simulink model "image_reject"  (R2014b)
settings: Solver=ode45  StartTime=0.0  StopTime=1  RelTol=1e-3
undefined symbols (not defined in the file or in its folder): fdesignblkfcn, gcbh
libraries: commrflib2 x1
settings Model: NumberOfSteps=100  Creator=Ben  LastModifiedBy=Ben

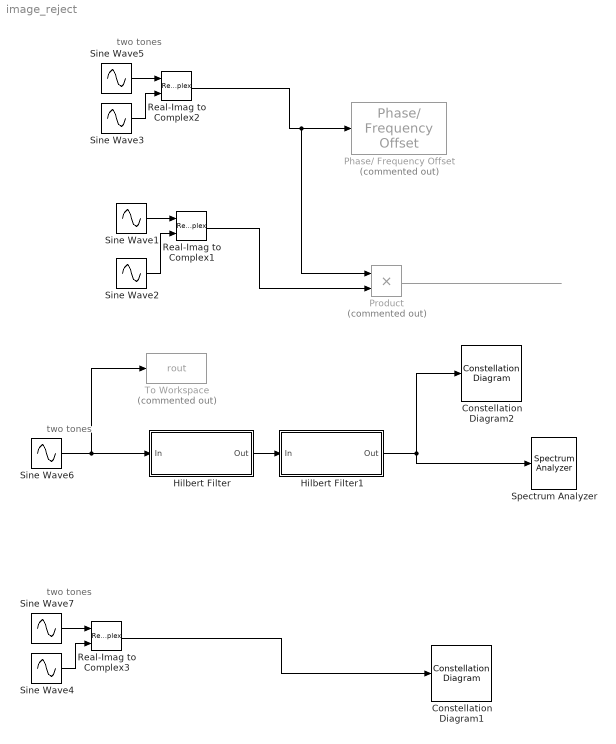
== system image_reject ==
  note: two tones
  note: two tones
  note: two tones
  Constellation Diagram1 : ConstellationDiagram
  Constellation Diagram2 : ConstellationDiagram
  Hilbert Filter : Subsystem  DialogController=fdesignblkfcn  InitFcn=fdesignblkfcn(gcbh, {'InitFcn'});  mask(Hilbert Filter){}
      mask help: Design a Hilbert filter
      settings: CopyFcn=fdesignblkfcn(gcbh, {'CopyFcn'});
      mask Help: helpview(mapfilelocation('dsp'), 'dsphilbertfilter');
      mask Display: disp('Hilbert')
  Hilbert Filter1 : Subsystem  DialogController=fdesignblkfcn  InitFcn=fdesignblkfcn(gcbh, {'InitFcn'});  mask(Hilbert Filter){}
      mask help: Design a Hilbert filter
      settings: CopyFcn=fdesignblkfcn(gcbh, {'CopyFcn'});
      mask Help: helpview(mapfilelocation('dsp'), 'dsphilbertfilter');
      mask Display: disp('Hilbert')
  Phase/ Frequency Offset : commrflib2/Phase// Frequency Offset  Commented=on  phaseOffset=0  freqPort=off  freqOffset=20000
  Product : Product  Commented=on
  Real-Imag to Complex1 : RealImagToComplex
  Real-Imag to Complex2 : RealImagToComplex
  Real-Imag to Complex3 : RealImagToComplex
  Sine Wave1 : Sin  Frequency=20000*2*pi  Phase=2*pi*90/360  SampleTime=2.00E-06
  Sine Wave2 : Sin  Frequency=20000*2*pi  SampleTime=2.00E-06
  Sine Wave{3..6} (4 alike) : Sin  Frequency=10*2*3.14*1000  SampleTime=2.00E-06
  Sine Wave7 : Sin  Frequency=10*2*3.14*1000  Phase=2*pi*90/360  SampleTime=2.00E-06
  Spectrum Analyzer : SpectrumAnalyzer
  To Workspace : ToWorkspace  Commented=on  VariableName=rout  SampleTime=-1
  wires:
  Sine Wave5/1 -> Real-Imag to Complex2/1
  Sine Wave1/1 -> Real-Imag to Complex1/1
  Real-Imag to Complex1/1 -> Product/2
  Real-Imag to Complex2/1 -> Product/1, Phase/ Frequency Offset/1
  Product/1 -> ?
  Sine Wave2/1 -> Real-Imag to Complex1/2
  Sine Wave3/1 -> Real-Imag to Complex2/2
  Sine Wave6/1 -> To Workspace/1, Hilbert Filter/1(In)
  Hilbert Filter/1(Out) -> Hilbert Filter1/1(In)
  Sine Wave7/1 -> Real-Imag to Complex3/1
  Sine Wave4/1 -> Real-Imag to Complex3/2
  Real-Imag to Complex3/1 -> Constellation Diagram1/1
  Hilbert Filter1/1(Out) -> Spectrum Analyzer/1, Constellation Diagram2/1

== system image_reject/Hilbert Filter ==
  In : Inport
  Generated Filter Block : Subsystem  Tag=FilterWizardSubSystem
  Out : Outport
  wires:
  Generated Filter Block/1(Output) -> Out/1
  In/1 -> Generated Filter Block/1(Input)

== system image_reject/Hilbert Filter1 ==
  In : Inport
  Generated Filter Block : Subsystem  Tag=FilterWizardSubSystem
  Out : Outport
  wires:
  Generated Filter Block/1(Output) -> Out/1
  In/1 -> Generated Filter Block/1(Input)

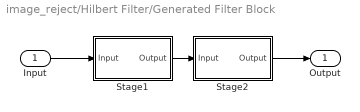
== system image_reject/Hilbert Filter/Generated Filter Block ==
  Input : Inport
  Stage1 : Subsystem  Tag=FilterWizardSubSystem
  Stage2 : Subsystem  Tag=FilterWizardSubSystem
      settings: ErrorFcn=dspFilterRealizedInBasicElemsAlgLoopErrFcnCallback
  Output : Outport
  wires:
  Input/1 -> Stage1/1(Input)
  Stage1/1(Output) -> Stage2/1(Input)
  Stage2/1(Output) -> Output/1

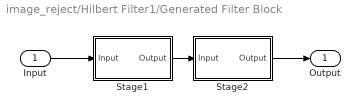
== system image_reject/Hilbert Filter1/Generated Filter Block ==
  Input : Inport
  Stage1 : Subsystem  Tag=FilterWizardSubSystem
  Stage2 : Subsystem  Tag=FilterWizardSubSystem
      settings: ErrorFcn=dspFilterRealizedInBasicElemsAlgLoopErrFcnCallback
  Output : Outport
  wires:
  Input/1 -> Stage1/1(Input)
  Stage1/1(Output) -> Stage2/1(Input)
  Stage2/1(Output) -> Output/1

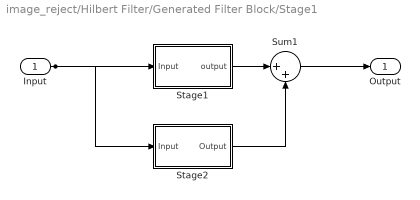
== system image_reject/Hilbert Filter/Generated Filter Block/Stage1 ==
  Input : Inport
  Stage1 : Subsystem  Tag=FilterWizardSubSystem
      settings: ErrorFcn=dspFilterRealizedInBasicElemsAlgLoopErrFcnCallback
  Stage2 : Subsystem  Tag=FilterWizardSubSystem
  Sum1 : Sum  Inputs=|++  RndMeth=Nearest  SaturateOnIntegerOverflow=on  OutDataTypeStr=Inherit: Same as first input
  Output : Outport
  wires:
  Stage1/1(output) -> Sum1/1
  Input/1 -> Stage1/1(Input), Stage2/1(Input)
  Stage2/1(Output) -> Sum1/2
  Sum1/1 -> Output/1

== system image_reject/Hilbert Filter/Generated Filter Block/Stage2 ==
  Input : Inport
  g(1) : Gain  Gain=0.5  ParamDataTypeStr=double  RndMeth=Nearest  SaturateOnIntegerOverflow=on  OutDataTypeStr=Inherit: Same as input
  Output : Outport
  wires:
  Input/1 -> g(1)/1
  g(1)/1 -> Output/1

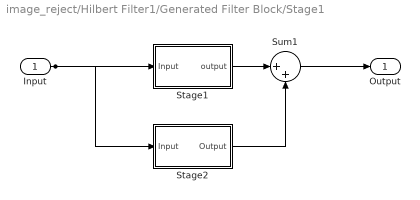
== system image_reject/Hilbert Filter1/Generated Filter Block/Stage1 ==
  Input : Inport
  Stage1 : Subsystem  Tag=FilterWizardSubSystem
      settings: ErrorFcn=dspFilterRealizedInBasicElemsAlgLoopErrFcnCallback
  Stage2 : Subsystem  Tag=FilterWizardSubSystem
  Sum1 : Sum  Inputs=|++  RndMeth=Nearest  SaturateOnIntegerOverflow=on  OutDataTypeStr=Inherit: Same as first input
  Output : Outport
  wires:
  Stage1/1(output) -> Sum1/1
  Input/1 -> Stage1/1(Input), Stage2/1(Input)
  Stage2/1(Output) -> Sum1/2
  Sum1/1 -> Output/1

== system image_reject/Hilbert Filter1/Generated Filter Block/Stage2 ==
  Input : Inport
  g(1) : Gain  Gain=0.5  ParamDataTypeStr=double  RndMeth=Nearest  SaturateOnIntegerOverflow=on  OutDataTypeStr=Inherit: Same as input
  Output : Outport
  wires:
  Input/1 -> g(1)/1
  g(1)/1 -> Output/1

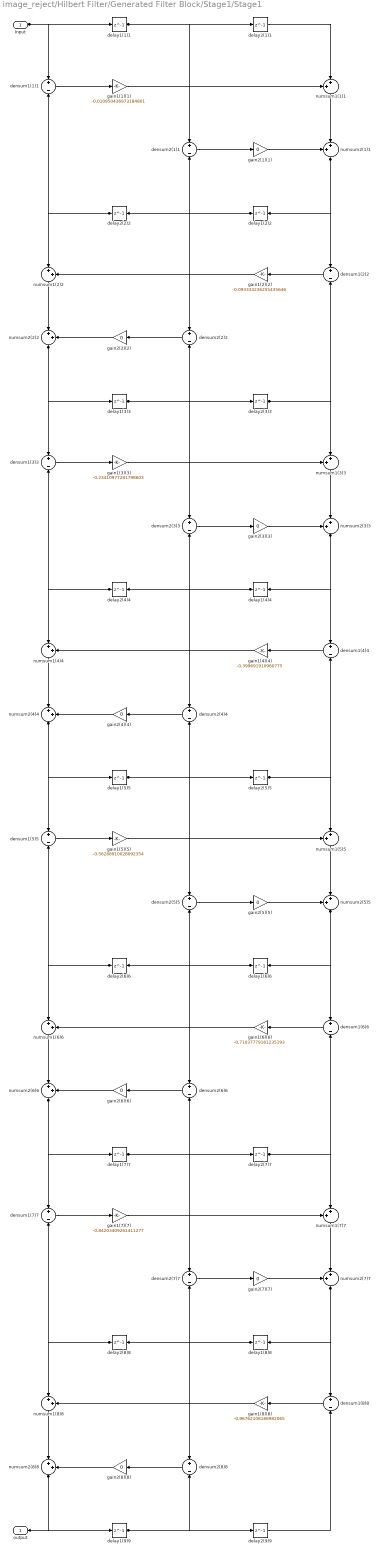
== system image_reject/Hilbert Filter/Generated Filter Block/Stage1/Stage1 ==
  Input : Inport
  delay1(1)1 : Delay  DelayLength=1  InitialCondition=0
  delay1(2)2 : Delay  DelayLength=1  InitialCondition=0
  delay1(3)3 : Delay  DelayLength=1  InitialCondition=0
  delay1(4)4 : Delay  DelayLength=1  InitialCondition=0
  delay1(5)5 : Delay  DelayLength=1  InitialCondition=0
  delay1(6)6 : Delay  DelayLength=1  InitialCondition=0
  delay1(7)7 : Delay  DelayLength=1  InitialCondition=0
  delay1(8)8 : Delay  DelayLength=1  InitialCondition=0
  delay1(9)9 : Delay  DelayLength=1  InitialCondition=0
  delay2(1)1 : Delay  DelayLength=1  InitialCondition=0
  delay2(2)2 : Delay  DelayLength=1  InitialCondition=0
  delay2(3)3 : Delay  DelayLength=1  InitialCondition=0
  delay2(4)4 : Delay  DelayLength=1  InitialCondition=0
  delay2(5)5 : Delay  DelayLength=1  InitialCondition=0
  delay2(6)6 : Delay  DelayLength=1  InitialCondition=0
  delay2(7)7 : Delay  DelayLength=1  InitialCondition=0
  delay2(8)8 : Delay  DelayLength=1  InitialCondition=0
  delay2(9)9 : Delay  DelayLength=1  InitialCondition=0
  densum1(1)1 : Sum  Inputs=+|-  RndMeth=Nearest  SaturateOnIntegerOverflow=on  OutDataTypeStr=Inherit: Same as first input
  densum1(2)2 : Sum  Inputs=+|-  RndMeth=Nearest  SaturateOnIntegerOverflow=on  OutDataTypeStr=Inherit: Same as first input
  densum1(3)3 : Sum  Inputs=+|-  RndMeth=Nearest  SaturateOnIntegerOverflow=on  OutDataTypeStr=Inherit: Same as first input
  densum1(4)4 : Sum  Inputs=+|-  RndMeth=Nearest  SaturateOnIntegerOverflow=on  OutDataTypeStr=Inherit: Same as first input
  densum1(5)5 : Sum  Inputs=+|-  RndMeth=Nearest  SaturateOnIntegerOverflow=on  OutDataTypeStr=Inherit: Same as first input
  densum1(6)6 : Sum  Inputs=+|-  RndMeth=Nearest  SaturateOnIntegerOverflow=on  OutDataTypeStr=Inherit: Same as first input
  densum1(7)7 : Sum  Inputs=+|-  RndMeth=Nearest  SaturateOnIntegerOverflow=on  OutDataTypeStr=Inherit: Same as first input
  densum1(8)8 : Sum  Inputs=+|-  RndMeth=Nearest  SaturateOnIntegerOverflow=on  OutDataTypeStr=Inherit: Same as first input
  densum2(1)1 : Sum  Inputs=+|-  RndMeth=Nearest  SaturateOnIntegerOverflow=on  OutDataTypeStr=Inherit: Same as first input
  densum2(2)2 : Sum  Inputs=+|-  RndMeth=Nearest  SaturateOnIntegerOverflow=on  OutDataTypeStr=Inherit: Same as first input
  densum2(3)3 : Sum  Inputs=+|-  RndMeth=Nearest  SaturateOnIntegerOverflow=on  OutDataTypeStr=Inherit: Same as first input
  densum2(4)4 : Sum  Inputs=+|-  RndMeth=Nearest  SaturateOnIntegerOverflow=on  OutDataTypeStr=Inherit: Same as first input
  densum2(5)5 : Sum  Inputs=+|-  RndMeth=Nearest  SaturateOnIntegerOverflow=on  OutDataTypeStr=Inherit: Same as first input
  densum2(6)6 : Sum  Inputs=+|-  RndMeth=Nearest  SaturateOnIntegerOverflow=on  OutDataTypeStr=Inherit: Same as first input
  densum2(7)7 : Sum  Inputs=+|-  RndMeth=Nearest  SaturateOnIntegerOverflow=on  OutDataTypeStr=Inherit: Same as first input
  densum2(8)8 : Sum  Inputs=+|-  RndMeth=Nearest  SaturateOnIntegerOverflow=on  OutDataTypeStr=Inherit: Same as first input
  gain1(1)(1) : Gain  Gain=-0.010950436973184801  ParamDataTypeStr=double  RndMeth=Nearest  SaturateOnIntegerOverflow=on  OutDataTypeStr=Inherit: Same as input
  gain1(2)(2) : Gain  Gain=-0.093334236255435646  ParamDataTypeStr=double  RndMeth=Nearest  SaturateOnIntegerOverflow=on  OutDataTypeStr=Inherit: Same as input
  gain1(3)(3) : Gain  Gain=-0.23410977281798603  ParamDataTypeStr=double  RndMeth=Nearest  SaturateOnIntegerOverflow=on  OutDataTypeStr=Inherit: Same as input
  gain1(4)(4) : Gain  Gain=-0.399691910960775  ParamDataTypeStr=double  RndMeth=Nearest  SaturateOnIntegerOverflow=on  OutDataTypeStr=Inherit: Same as input
  gain1(5)(5) : Gain  Gain=-0.56288910028092354  ParamDataTypeStr=double  RndMeth=Nearest  SaturateOnIntegerOverflow=on  OutDataTypeStr=Inherit: Same as input
  gain1(6)(6) : Gain  Gain=-0.71037779161235193  ParamDataTypeStr=double  RndMeth=Nearest  SaturateOnIntegerOverflow=on  OutDataTypeStr=Inherit: Same as input
  gain1(7)(7) : Gain  Gain=-0.84203409261411277  ParamDataTypeStr=double  RndMeth=Nearest  SaturateOnIntegerOverflow=on  OutDataTypeStr=Inherit: Same as input
  gain1(8)(8) : Gain  Gain=-0.96762108186982065  ParamDataTypeStr=double  RndMeth=Nearest  SaturateOnIntegerOverflow=on  OutDataTypeStr=Inherit: Same as input
  gain2(1)(1) : Gain  Gain=0  ParamDataTypeStr=double  RndMeth=Nearest  SaturateOnIntegerOverflow=on  OutDataTypeStr=Inherit: Same as input
  gain2(2)(2) : Gain  Gain=0  ParamDataTypeStr=double  RndMeth=Nearest  SaturateOnIntegerOverflow=on  OutDataTypeStr=Inherit: Same as input
  gain2(3)(3) : Gain  Gain=0  ParamDataTypeStr=double  RndMeth=Nearest  SaturateOnIntegerOverflow=on  OutDataTypeStr=Inherit: Same as input
  gain2(4)(4) : Gain  Gain=0  ParamDataTypeStr=double  RndMeth=Nearest  SaturateOnIntegerOverflow=on  OutDataTypeStr=Inherit: Same as input
  gain2(5)(5) : Gain  Gain=0  ParamDataTypeStr=double  RndMeth=Nearest  SaturateOnIntegerOverflow=on  OutDataTypeStr=Inherit: Same as input
  gain2(6)(6) : Gain  Gain=0  ParamDataTypeStr=double  RndMeth=Nearest  SaturateOnIntegerOverflow=on  OutDataTypeStr=Inherit: Same as input
  gain2(7)(7) : Gain  Gain=0  ParamDataTypeStr=double  RndMeth=Nearest  SaturateOnIntegerOverflow=on  OutDataTypeStr=Inherit: Same as input
  gain2(8)(8) : Gain  Gain=0  ParamDataTypeStr=double  RndMeth=Nearest  SaturateOnIntegerOverflow=on  OutDataTypeStr=Inherit: Same as input
  numsum1(1)1 : Sum  Inputs=++|  RndMeth=Nearest  SaturateOnIntegerOverflow=on  OutDataTypeStr=Inherit: Same as first input
  numsum1(2)2 : Sum  Inputs=|++  RndMeth=Nearest  SaturateOnIntegerOverflow=on  OutDataTypeStr=Inherit: Same as first input
  numsum1(3)3 : Sum  Inputs=++|  RndMeth=Nearest  SaturateOnIntegerOverflow=on  OutDataTypeStr=Inherit: Same as first input
  numsum1(4)4 : Sum  Inputs=|++  RndMeth=Nearest  SaturateOnIntegerOverflow=on  OutDataTypeStr=Inherit: Same as first input
  numsum1(5)5 : Sum  Inputs=++|  RndMeth=Nearest  SaturateOnIntegerOverflow=on  OutDataTypeStr=Inherit: Same as first input
  numsum1(6)6 : Sum  Inputs=|++  RndMeth=Nearest  SaturateOnIntegerOverflow=on  OutDataTypeStr=Inherit: Same as first input
  numsum1(7)7 : Sum  Inputs=++|  RndMeth=Nearest  SaturateOnIntegerOverflow=on  OutDataTypeStr=Inherit: Same as first input
  numsum1(8)8 : Sum  Inputs=|++  RndMeth=Nearest  SaturateOnIntegerOverflow=on  OutDataTypeStr=Inherit: Same as first input
  numsum2(1)1 : Sum  Inputs=++|  RndMeth=Nearest  SaturateOnIntegerOverflow=on  OutDataTypeStr=Inherit: Same as first input
  numsum2(2)2 : Sum  Inputs=|++  RndMeth=Nearest  SaturateOnIntegerOverflow=on  OutDataTypeStr=Inherit: Same as first input
  numsum2(3)3 : Sum  Inputs=++|  RndMeth=Nearest  SaturateOnIntegerOverflow=on  OutDataTypeStr=Inherit: Same as first input
  numsum2(4)4 : Sum  Inputs=|++  RndMeth=Nearest  SaturateOnIntegerOverflow=on  OutDataTypeStr=Inherit: Same as first input
  numsum2(5)5 : Sum  Inputs=++|  RndMeth=Nearest  SaturateOnIntegerOverflow=on  OutDataTypeStr=Inherit: Same as first input
  numsum2(6)6 : Sum  Inputs=|++  RndMeth=Nearest  SaturateOnIntegerOverflow=on  OutDataTypeStr=Inherit: Same as first input
  numsum2(7)7 : Sum  Inputs=++|  RndMeth=Nearest  SaturateOnIntegerOverflow=on  OutDataTypeStr=Inherit: Same as first input
  numsum2(8)8 : Sum  Inputs=|++  RndMeth=Nearest  SaturateOnIntegerOverflow=on  OutDataTypeStr=Inherit: Same as first input
  output : Outport
  wires:
  delay1(1)1/1 -> delay2(1)1/1, densum2(1)1/1
  delay2(1)1/1 -> numsum1(1)1/2
  densum1(1)1/1 -> gain1(1)(1)/1
  gain1(1)(1)/1 -> numsum1(1)1/1
  numsum1(1)1/1 -> numsum2(1)1/2
  densum2(1)1/1 -> gain2(1)(1)/1
  gain2(1)(1)/1 -> numsum2(1)1/1
  numsum2(1)1/1 -> delay1(2)2/1, densum1(2)2/1
  Input/1 -> delay1(1)1/1, densum1(1)1/1
  delay1(2)2/1 -> delay2(2)2/1, densum2(2)2/1, densum2(1)1/2
  delay2(2)2/1 -> numsum1(2)2/1, densum1(1)1/2
  densum1(2)2/1 -> gain1(2)(2)/1
  gain1(2)(2)/1 -> numsum1(2)2/2
  numsum1(2)2/1 -> numsum2(2)2/1
  densum2(2)2/1 -> gain2(2)(2)/1
  gain2(2)(2)/1 -> numsum2(2)2/2
  numsum2(2)2/1 -> delay1(3)3/1, densum1(3)3/1
  delay1(3)3/1 -> delay2(3)3/1, densum2(3)3/1, densum2(2)2/2
  delay2(3)3/1 -> numsum1(3)3/2, densum1(2)2/2
  densum1(3)3/1 -> gain1(3)(3)/1
  gain1(3)(3)/1 -> numsum1(3)3/1
  numsum1(3)3/1 -> numsum2(3)3/2
  densum2(3)3/1 -> gain2(3)(3)/1
  gain2(3)(3)/1 -> numsum2(3)3/1
  numsum2(3)3/1 -> delay1(4)4/1, densum1(4)4/1
  delay1(4)4/1 -> delay2(4)4/1, densum2(4)4/1, densum2(3)3/2
  delay2(4)4/1 -> numsum1(4)4/1, densum1(3)3/2
  densum1(4)4/1 -> gain1(4)(4)/1
  gain1(4)(4)/1 -> numsum1(4)4/2
  numsum1(4)4/1 -> numsum2(4)4/1
  densum2(4)4/1 -> gain2(4)(4)/1
  gain2(4)(4)/1 -> numsum2(4)4/2
  numsum2(4)4/1 -> delay1(5)5/1, densum1(5)5/1
  delay1(5)5/1 -> delay2(5)5/1, densum2(5)5/1, densum2(4)4/2
  delay2(5)5/1 -> numsum1(5)5/2, densum1(4)4/2
  densum1(5)5/1 -> gain1(5)(5)/1
  gain1(5)(5)/1 -> numsum1(5)5/1
  numsum1(5)5/1 -> numsum2(5)5/2
  densum2(5)5/1 -> gain2(5)(5)/1
  gain2(5)(5)/1 -> numsum2(5)5/1
  numsum2(5)5/1 -> delay1(6)6/1, densum1(6)6/1
  delay1(6)6/1 -> delay2(6)6/1, densum2(6)6/1, densum2(5)5/2
  delay2(6)6/1 -> numsum1(6)6/1, densum1(5)5/2
  densum1(6)6/1 -> gain1(6)(6)/1
  gain1(6)(6)/1 -> numsum1(6)6/2
  numsum1(6)6/1 -> numsum2(6)6/1
  densum2(6)6/1 -> gain2(6)(6)/1
  gain2(6)(6)/1 -> numsum2(6)6/2
  numsum2(6)6/1 -> delay1(7)7/1, densum1(7)7/1
  delay1(7)7/1 -> delay2(7)7/1, densum2(7)7/1, densum2(6)6/2
  delay2(7)7/1 -> numsum1(7)7/2, densum1(6)6/2
  densum1(7)7/1 -> gain1(7)(7)/1
  gain1(7)(7)/1 -> numsum1(7)7/1
  numsum1(7)7/1 -> numsum2(7)7/2
  densum2(7)7/1 -> gain2(7)(7)/1
  gain2(7)(7)/1 -> numsum2(7)7/1
  numsum2(7)7/1 -> delay1(8)8/1, densum1(8)8/1
  delay1(8)8/1 -> delay2(8)8/1, densum2(8)8/1, densum2(7)7/2
  delay2(8)8/1 -> numsum1(8)8/1, densum1(7)7/2
  densum1(8)8/1 -> gain1(8)(8)/1
  gain1(8)(8)/1 -> numsum1(8)8/2
  numsum1(8)8/1 -> numsum2(8)8/1
  densum2(8)8/1 -> gain2(8)(8)/1
  gain2(8)(8)/1 -> numsum2(8)8/2
  numsum2(8)8/1 -> delay1(9)9/1, output/1
  delay1(9)9/1 -> delay2(9)9/1, densum2(8)8/2
  delay2(9)9/1 -> densum1(8)8/2

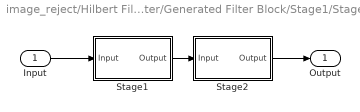
== system image_reject/Hilbert Filter/Generated Filter Block/Stage1/Stage2 ==
  Input : Inport
  Stage1 : Subsystem  Tag=FilterWizardSubSystem
      settings: ErrorFcn=dspFilterRealizedInBasicElemsAlgLoopErrFcnCallback
  Stage2 : Subsystem  Tag=FilterWizardSubSystem
  Output : Outport
  wires:
  Input/1 -> Stage1/1(Input)
  Stage1/1(Output) -> Stage2/1(Input)
  Stage2/1(Output) -> Output/1

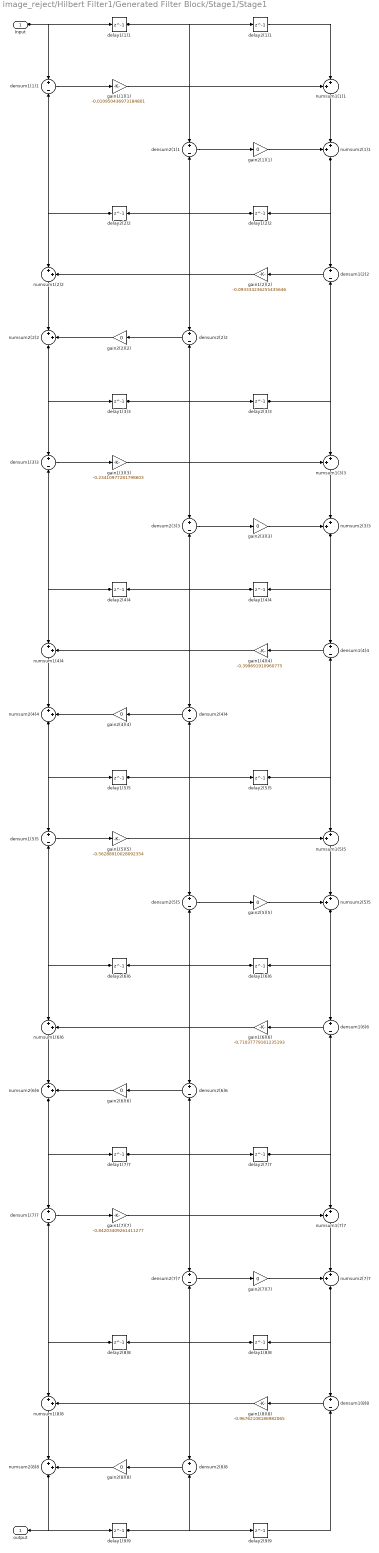
== system image_reject/Hilbert Filter1/Generated Filter Block/Stage1/Stage1 ==
  Input : Inport
  delay1(1)1 : Delay  DelayLength=1  InitialCondition=0
  delay1(2)2 : Delay  DelayLength=1  InitialCondition=0
  delay1(3)3 : Delay  DelayLength=1  InitialCondition=0
  delay1(4)4 : Delay  DelayLength=1  InitialCondition=0
  delay1(5)5 : Delay  DelayLength=1  InitialCondition=0
  delay1(6)6 : Delay  DelayLength=1  InitialCondition=0
  delay1(7)7 : Delay  DelayLength=1  InitialCondition=0
  delay1(8)8 : Delay  DelayLength=1  InitialCondition=0
  delay1(9)9 : Delay  DelayLength=1  InitialCondition=0
  delay2(1)1 : Delay  DelayLength=1  InitialCondition=0
  delay2(2)2 : Delay  DelayLength=1  InitialCondition=0
  delay2(3)3 : Delay  DelayLength=1  InitialCondition=0
  delay2(4)4 : Delay  DelayLength=1  InitialCondition=0
  delay2(5)5 : Delay  DelayLength=1  InitialCondition=0
  delay2(6)6 : Delay  DelayLength=1  InitialCondition=0
  delay2(7)7 : Delay  DelayLength=1  InitialCondition=0
  delay2(8)8 : Delay  DelayLength=1  InitialCondition=0
  delay2(9)9 : Delay  DelayLength=1  InitialCondition=0
  densum1(1)1 : Sum  Inputs=+|-  RndMeth=Nearest  SaturateOnIntegerOverflow=on  OutDataTypeStr=Inherit: Same as first input
  densum1(2)2 : Sum  Inputs=+|-  RndMeth=Nearest  SaturateOnIntegerOverflow=on  OutDataTypeStr=Inherit: Same as first input
  densum1(3)3 : Sum  Inputs=+|-  RndMeth=Nearest  SaturateOnIntegerOverflow=on  OutDataTypeStr=Inherit: Same as first input
  densum1(4)4 : Sum  Inputs=+|-  RndMeth=Nearest  SaturateOnIntegerOverflow=on  OutDataTypeStr=Inherit: Same as first input
  densum1(5)5 : Sum  Inputs=+|-  RndMeth=Nearest  SaturateOnIntegerOverflow=on  OutDataTypeStr=Inherit: Same as first input
  densum1(6)6 : Sum  Inputs=+|-  RndMeth=Nearest  SaturateOnIntegerOverflow=on  OutDataTypeStr=Inherit: Same as first input
  densum1(7)7 : Sum  Inputs=+|-  RndMeth=Nearest  SaturateOnIntegerOverflow=on  OutDataTypeStr=Inherit: Same as first input
  densum1(8)8 : Sum  Inputs=+|-  RndMeth=Nearest  SaturateOnIntegerOverflow=on  OutDataTypeStr=Inherit: Same as first input
  densum2(1)1 : Sum  Inputs=+|-  RndMeth=Nearest  SaturateOnIntegerOverflow=on  OutDataTypeStr=Inherit: Same as first input
  densum2(2)2 : Sum  Inputs=+|-  RndMeth=Nearest  SaturateOnIntegerOverflow=on  OutDataTypeStr=Inherit: Same as first input
  densum2(3)3 : Sum  Inputs=+|-  RndMeth=Nearest  SaturateOnIntegerOverflow=on  OutDataTypeStr=Inherit: Same as first input
  densum2(4)4 : Sum  Inputs=+|-  RndMeth=Nearest  SaturateOnIntegerOverflow=on  OutDataTypeStr=Inherit: Same as first input
  densum2(5)5 : Sum  Inputs=+|-  RndMeth=Nearest  SaturateOnIntegerOverflow=on  OutDataTypeStr=Inherit: Same as first input
  densum2(6)6 : Sum  Inputs=+|-  RndMeth=Nearest  SaturateOnIntegerOverflow=on  OutDataTypeStr=Inherit: Same as first input
  densum2(7)7 : Sum  Inputs=+|-  RndMeth=Nearest  SaturateOnIntegerOverflow=on  OutDataTypeStr=Inherit: Same as first input
  densum2(8)8 : Sum  Inputs=+|-  RndMeth=Nearest  SaturateOnIntegerOverflow=on  OutDataTypeStr=Inherit: Same as first input
  gain1(1)(1) : Gain  Gain=-0.010950436973184801  ParamDataTypeStr=double  RndMeth=Nearest  SaturateOnIntegerOverflow=on  OutDataTypeStr=Inherit: Same as input
  gain1(2)(2) : Gain  Gain=-0.093334236255435646  ParamDataTypeStr=double  RndMeth=Nearest  SaturateOnIntegerOverflow=on  OutDataTypeStr=Inherit: Same as input
  gain1(3)(3) : Gain  Gain=-0.23410977281798603  ParamDataTypeStr=double  RndMeth=Nearest  SaturateOnIntegerOverflow=on  OutDataTypeStr=Inherit: Same as input
  gain1(4)(4) : Gain  Gain=-0.399691910960775  ParamDataTypeStr=double  RndMeth=Nearest  SaturateOnIntegerOverflow=on  OutDataTypeStr=Inherit: Same as input
  gain1(5)(5) : Gain  Gain=-0.56288910028092354  ParamDataTypeStr=double  RndMeth=Nearest  SaturateOnIntegerOverflow=on  OutDataTypeStr=Inherit: Same as input
  gain1(6)(6) : Gain  Gain=-0.71037779161235193  ParamDataTypeStr=double  RndMeth=Nearest  SaturateOnIntegerOverflow=on  OutDataTypeStr=Inherit: Same as input
  gain1(7)(7) : Gain  Gain=-0.84203409261411277  ParamDataTypeStr=double  RndMeth=Nearest  SaturateOnIntegerOverflow=on  OutDataTypeStr=Inherit: Same as input
  gain1(8)(8) : Gain  Gain=-0.96762108186982065  ParamDataTypeStr=double  RndMeth=Nearest  SaturateOnIntegerOverflow=on  OutDataTypeStr=Inherit: Same as input
  gain2(1)(1) : Gain  Gain=0  ParamDataTypeStr=double  RndMeth=Nearest  SaturateOnIntegerOverflow=on  OutDataTypeStr=Inherit: Same as input
  gain2(2)(2) : Gain  Gain=0  ParamDataTypeStr=double  RndMeth=Nearest  SaturateOnIntegerOverflow=on  OutDataTypeStr=Inherit: Same as input
  gain2(3)(3) : Gain  Gain=0  ParamDataTypeStr=double  RndMeth=Nearest  SaturateOnIntegerOverflow=on  OutDataTypeStr=Inherit: Same as input
  gain2(4)(4) : Gain  Gain=0  ParamDataTypeStr=double  RndMeth=Nearest  SaturateOnIntegerOverflow=on  OutDataTypeStr=Inherit: Same as input
  gain2(5)(5) : Gain  Gain=0  ParamDataTypeStr=double  RndMeth=Nearest  SaturateOnIntegerOverflow=on  OutDataTypeStr=Inherit: Same as input
  gain2(6)(6) : Gain  Gain=0  ParamDataTypeStr=double  RndMeth=Nearest  SaturateOnIntegerOverflow=on  OutDataTypeStr=Inherit: Same as input
  gain2(7)(7) : Gain  Gain=0  ParamDataTypeStr=double  RndMeth=Nearest  SaturateOnIntegerOverflow=on  OutDataTypeStr=Inherit: Same as input
  gain2(8)(8) : Gain  Gain=0  ParamDataTypeStr=double  RndMeth=Nearest  SaturateOnIntegerOverflow=on  OutDataTypeStr=Inherit: Same as input
  numsum1(1)1 : Sum  Inputs=++|  RndMeth=Nearest  SaturateOnIntegerOverflow=on  OutDataTypeStr=Inherit: Same as first input
  numsum1(2)2 : Sum  Inputs=|++  RndMeth=Nearest  SaturateOnIntegerOverflow=on  OutDataTypeStr=Inherit: Same as first input
  numsum1(3)3 : Sum  Inputs=++|  RndMeth=Nearest  SaturateOnIntegerOverflow=on  OutDataTypeStr=Inherit: Same as first input
  numsum1(4)4 : Sum  Inputs=|++  RndMeth=Nearest  SaturateOnIntegerOverflow=on  OutDataTypeStr=Inherit: Same as first input
  numsum1(5)5 : Sum  Inputs=++|  RndMeth=Nearest  SaturateOnIntegerOverflow=on  OutDataTypeStr=Inherit: Same as first input
  numsum1(6)6 : Sum  Inputs=|++  RndMeth=Nearest  SaturateOnIntegerOverflow=on  OutDataTypeStr=Inherit: Same as first input
  numsum1(7)7 : Sum  Inputs=++|  RndMeth=Nearest  SaturateOnIntegerOverflow=on  OutDataTypeStr=Inherit: Same as first input
  numsum1(8)8 : Sum  Inputs=|++  RndMeth=Nearest  SaturateOnIntegerOverflow=on  OutDataTypeStr=Inherit: Same as first input
  numsum2(1)1 : Sum  Inputs=++|  RndMeth=Nearest  SaturateOnIntegerOverflow=on  OutDataTypeStr=Inherit: Same as first input
  numsum2(2)2 : Sum  Inputs=|++  RndMeth=Nearest  SaturateOnIntegerOverflow=on  OutDataTypeStr=Inherit: Same as first input
  numsum2(3)3 : Sum  Inputs=++|  RndMeth=Nearest  SaturateOnIntegerOverflow=on  OutDataTypeStr=Inherit: Same as first input
  numsum2(4)4 : Sum  Inputs=|++  RndMeth=Nearest  SaturateOnIntegerOverflow=on  OutDataTypeStr=Inherit: Same as first input
  numsum2(5)5 : Sum  Inputs=++|  RndMeth=Nearest  SaturateOnIntegerOverflow=on  OutDataTypeStr=Inherit: Same as first input
  numsum2(6)6 : Sum  Inputs=|++  RndMeth=Nearest  SaturateOnIntegerOverflow=on  OutDataTypeStr=Inherit: Same as first input
  numsum2(7)7 : Sum  Inputs=++|  RndMeth=Nearest  SaturateOnIntegerOverflow=on  OutDataTypeStr=Inherit: Same as first input
  numsum2(8)8 : Sum  Inputs=|++  RndMeth=Nearest  SaturateOnIntegerOverflow=on  OutDataTypeStr=Inherit: Same as first input
  output : Outport
  wires:
  delay1(1)1/1 -> delay2(1)1/1, densum2(1)1/1
  delay2(1)1/1 -> numsum1(1)1/2
  densum1(1)1/1 -> gain1(1)(1)/1
  gain1(1)(1)/1 -> numsum1(1)1/1
  numsum1(1)1/1 -> numsum2(1)1/2
  densum2(1)1/1 -> gain2(1)(1)/1
  gain2(1)(1)/1 -> numsum2(1)1/1
  numsum2(1)1/1 -> delay1(2)2/1, densum1(2)2/1
  Input/1 -> delay1(1)1/1, densum1(1)1/1
  delay1(2)2/1 -> delay2(2)2/1, densum2(2)2/1, densum2(1)1/2
  delay2(2)2/1 -> numsum1(2)2/1, densum1(1)1/2
  densum1(2)2/1 -> gain1(2)(2)/1
  gain1(2)(2)/1 -> numsum1(2)2/2
  numsum1(2)2/1 -> numsum2(2)2/1
  densum2(2)2/1 -> gain2(2)(2)/1
  gain2(2)(2)/1 -> numsum2(2)2/2
  numsum2(2)2/1 -> delay1(3)3/1, densum1(3)3/1
  delay1(3)3/1 -> delay2(3)3/1, densum2(3)3/1, densum2(2)2/2
  delay2(3)3/1 -> numsum1(3)3/2, densum1(2)2/2
  densum1(3)3/1 -> gain1(3)(3)/1
  gain1(3)(3)/1 -> numsum1(3)3/1
  numsum1(3)3/1 -> numsum2(3)3/2
  densum2(3)3/1 -> gain2(3)(3)/1
  gain2(3)(3)/1 -> numsum2(3)3/1
  numsum2(3)3/1 -> delay1(4)4/1, densum1(4)4/1
  delay1(4)4/1 -> delay2(4)4/1, densum2(4)4/1, densum2(3)3/2
  delay2(4)4/1 -> numsum1(4)4/1, densum1(3)3/2
  densum1(4)4/1 -> gain1(4)(4)/1
  gain1(4)(4)/1 -> numsum1(4)4/2
  numsum1(4)4/1 -> numsum2(4)4/1
  densum2(4)4/1 -> gain2(4)(4)/1
  gain2(4)(4)/1 -> numsum2(4)4/2
  numsum2(4)4/1 -> delay1(5)5/1, densum1(5)5/1
  delay1(5)5/1 -> delay2(5)5/1, densum2(5)5/1, densum2(4)4/2
  delay2(5)5/1 -> numsum1(5)5/2, densum1(4)4/2
  densum1(5)5/1 -> gain1(5)(5)/1
  gain1(5)(5)/1 -> numsum1(5)5/1
  numsum1(5)5/1 -> numsum2(5)5/2
  densum2(5)5/1 -> gain2(5)(5)/1
  gain2(5)(5)/1 -> numsum2(5)5/1
  numsum2(5)5/1 -> delay1(6)6/1, densum1(6)6/1
  delay1(6)6/1 -> delay2(6)6/1, densum2(6)6/1, densum2(5)5/2
  delay2(6)6/1 -> numsum1(6)6/1, densum1(5)5/2
  densum1(6)6/1 -> gain1(6)(6)/1
  gain1(6)(6)/1 -> numsum1(6)6/2
  numsum1(6)6/1 -> numsum2(6)6/1
  densum2(6)6/1 -> gain2(6)(6)/1
  gain2(6)(6)/1 -> numsum2(6)6/2
  numsum2(6)6/1 -> delay1(7)7/1, densum1(7)7/1
  delay1(7)7/1 -> delay2(7)7/1, densum2(7)7/1, densum2(6)6/2
  delay2(7)7/1 -> numsum1(7)7/2, densum1(6)6/2
  densum1(7)7/1 -> gain1(7)(7)/1
  gain1(7)(7)/1 -> numsum1(7)7/1
  numsum1(7)7/1 -> numsum2(7)7/2
  densum2(7)7/1 -> gain2(7)(7)/1
  gain2(7)(7)/1 -> numsum2(7)7/1
  numsum2(7)7/1 -> delay1(8)8/1, densum1(8)8/1
  delay1(8)8/1 -> delay2(8)8/1, densum2(8)8/1, densum2(7)7/2
  delay2(8)8/1 -> numsum1(8)8/1, densum1(7)7/2
  densum1(8)8/1 -> gain1(8)(8)/1
  gain1(8)(8)/1 -> numsum1(8)8/2
  numsum1(8)8/1 -> numsum2(8)8/1
  densum2(8)8/1 -> gain2(8)(8)/1
  gain2(8)(8)/1 -> numsum2(8)8/2
  numsum2(8)8/1 -> delay1(9)9/1, output/1
  delay1(9)9/1 -> delay2(9)9/1, densum2(8)8/2
  delay2(9)9/1 -> densum1(8)8/2

== system image_reject/Hilbert Filter1/Generated Filter Block/Stage1/Stage2 ==
  Input : Inport
  Stage1 : Subsystem  Tag=FilterWizardSubSystem
      settings: ErrorFcn=dspFilterRealizedInBasicElemsAlgLoopErrFcnCallback
  Stage2 : Subsystem  Tag=FilterWizardSubSystem
  Output : Outport
  wires:
  Input/1 -> Stage1/1(Input)
  Stage1/1(Output) -> Stage2/1(Input)
  Stage2/1(Output) -> Output/1

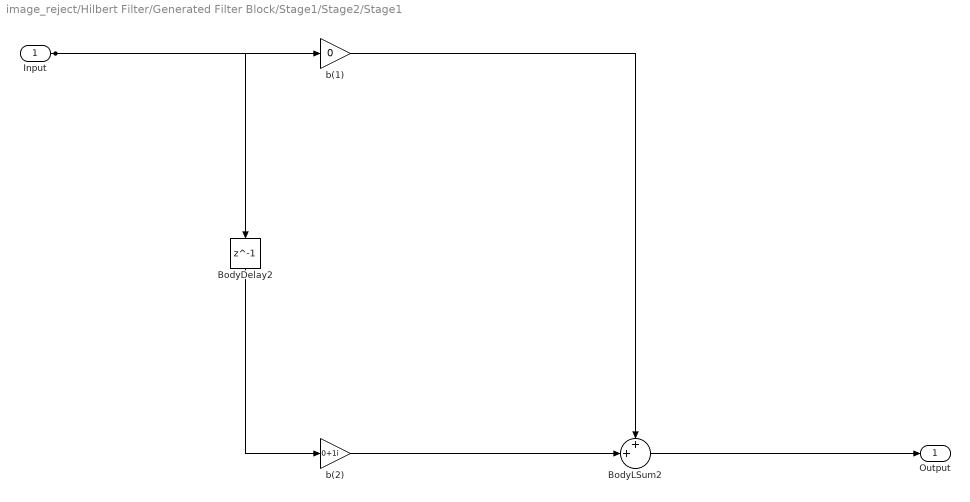
== system image_reject/Hilbert Filter/Generated Filter Block/Stage1/Stage2/Stage1 ==
  Input : Inport
  BodyDelay2 : Delay  DelayLength=1  InitialCondition=0
  BodyLSum2 : Sum  Inputs=++|  RndMeth=Nearest  SaturateOnIntegerOverflow=on  OutDataTypeStr=Inherit: Same as first input
  b(1) : Gain  Gain=0  ParamDataTypeStr=double  RndMeth=Nearest  SaturateOnIntegerOverflow=on  OutDataTypeStr=Inherit: Same as input
  b(2) : Gain  Gain=0+1i  ParamDataTypeStr=double  RndMeth=Nearest  SaturateOnIntegerOverflow=on  OutDataTypeStr=Inherit: Same as input
  Output : Outport
  wires:
  Input/1 -> b(1)/1, BodyDelay2/1
  b(1)/1 -> BodyLSum2/1
  BodyDelay2/1 -> b(2)/1
  b(2)/1 -> BodyLSum2/2
  BodyLSum2/1 -> Output/1

== system image_reject/Hilbert Filter/Generated Filter Block/Stage1/Stage2/Stage2 ==
  Input : Inport
  Stage1 : Subsystem  Tag=FilterWizardSubSystem
      settings: ErrorFcn=dspFilterRealizedInBasicElemsAlgLoopErrFcnCallback
  Stage2 : Subsystem  Tag=FilterWizardSubSystem
      settings: ErrorFcn=dspFilterRealizedInBasicElemsAlgLoopErrFcnCallback
  Output : Outport
  wires:
  Input/1 -> Stage1/1(Input)
  Stage1/1(Output) -> Stage2/1(Input)
  Stage2/1(output) -> Output/1

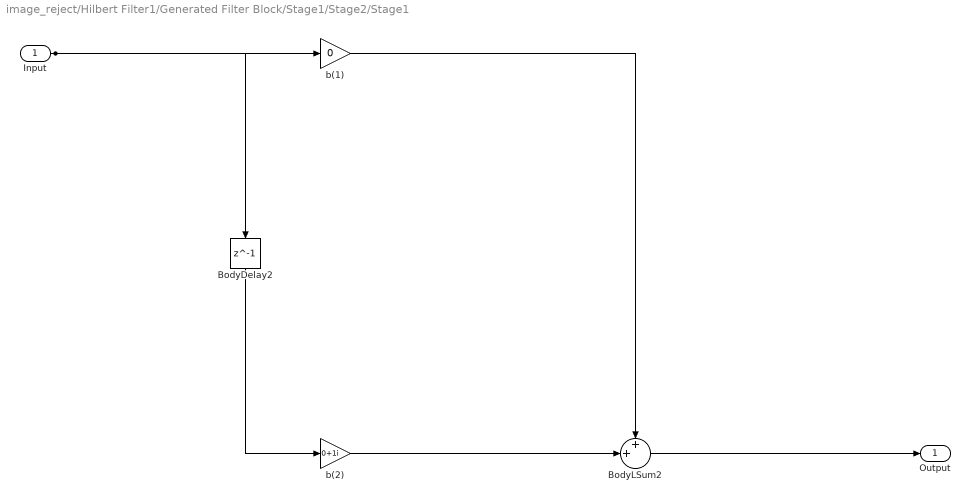
== system image_reject/Hilbert Filter1/Generated Filter Block/Stage1/Stage2/Stage1 ==
  Input : Inport
  BodyDelay2 : Delay  DelayLength=1  InitialCondition=0
  BodyLSum2 : Sum  Inputs=++|  RndMeth=Nearest  SaturateOnIntegerOverflow=on  OutDataTypeStr=Inherit: Same as first input
  b(1) : Gain  Gain=0  ParamDataTypeStr=double  RndMeth=Nearest  SaturateOnIntegerOverflow=on  OutDataTypeStr=Inherit: Same as input
  b(2) : Gain  Gain=0+1i  ParamDataTypeStr=double  RndMeth=Nearest  SaturateOnIntegerOverflow=on  OutDataTypeStr=Inherit: Same as input
  Output : Outport
  wires:
  Input/1 -> b(1)/1, BodyDelay2/1
  b(1)/1 -> BodyLSum2/1
  BodyDelay2/1 -> b(2)/1
  b(2)/1 -> BodyLSum2/2
  BodyLSum2/1 -> Output/1

== system image_reject/Hilbert Filter1/Generated Filter Block/Stage1/Stage2/Stage2 ==
  Input : Inport
  Stage1 : Subsystem  Tag=FilterWizardSubSystem
      settings: ErrorFcn=dspFilterRealizedInBasicElemsAlgLoopErrFcnCallback
  Stage2 : Subsystem  Tag=FilterWizardSubSystem
      settings: ErrorFcn=dspFilterRealizedInBasicElemsAlgLoopErrFcnCallback
  Output : Outport
  wires:
  Input/1 -> Stage1/1(Input)
  Stage1/1(Output) -> Stage2/1(Input)
  Stage2/1(output) -> Output/1

== system image_reject/Hilbert Filter/Generated Filter Block/Stage1/Stage2/Stage2/Stage1 ==
  Input : Inport
  g(1) : Gain  Gain=-1  ParamDataTypeStr=double  RndMeth=Nearest  SaturateOnIntegerOverflow=on  OutDataTypeStr=Inherit: Same as input
  Output : Outport
  wires:
  Input/1 -> g(1)/1
  g(1)/1 -> Output/1

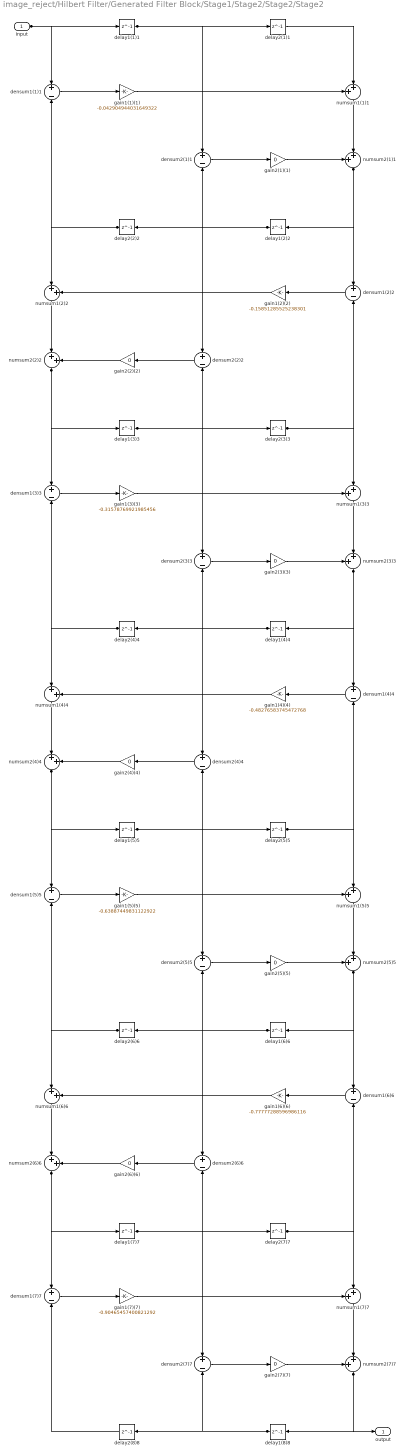
== system image_reject/Hilbert Filter/Generated Filter Block/Stage1/Stage2/Stage2/Stage2 ==
  Input : Inport
  delay1(1)1 : Delay  DelayLength=1  InitialCondition=0
  delay1(2)2 : Delay  DelayLength=1  InitialCondition=0
  delay1(3)3 : Delay  DelayLength=1  InitialCondition=0
  delay1(4)4 : Delay  DelayLength=1  InitialCondition=0
  delay1(5)5 : Delay  DelayLength=1  InitialCondition=0
  delay1(6)6 : Delay  DelayLength=1  InitialCondition=0
  delay1(7)7 : Delay  DelayLength=1  InitialCondition=0
  delay1(8)8 : Delay  DelayLength=1  InitialCondition=0
  delay2(1)1 : Delay  DelayLength=1  InitialCondition=0
  delay2(2)2 : Delay  DelayLength=1  InitialCondition=0
  delay2(3)3 : Delay  DelayLength=1  InitialCondition=0
  delay2(4)4 : Delay  DelayLength=1  InitialCondition=0
  delay2(5)5 : Delay  DelayLength=1  InitialCondition=0
  delay2(6)6 : Delay  DelayLength=1  InitialCondition=0
  delay2(7)7 : Delay  DelayLength=1  InitialCondition=0
  delay2(8)8 : Delay  DelayLength=1  InitialCondition=0
  densum1(1)1 : Sum  Inputs=+|-  RndMeth=Nearest  SaturateOnIntegerOverflow=on  OutDataTypeStr=Inherit: Same as first input
  densum1(2)2 : Sum  Inputs=+|-  RndMeth=Nearest  SaturateOnIntegerOverflow=on  OutDataTypeStr=Inherit: Same as first input
  densum1(3)3 : Sum  Inputs=+|-  RndMeth=Nearest  SaturateOnIntegerOverflow=on  OutDataTypeStr=Inherit: Same as first input
  densum1(4)4 : Sum  Inputs=+|-  RndMeth=Nearest  SaturateOnIntegerOverflow=on  OutDataTypeStr=Inherit: Same as first input
  densum1(5)5 : Sum  Inputs=+|-  RndMeth=Nearest  SaturateOnIntegerOverflow=on  OutDataTypeStr=Inherit: Same as first input
  densum1(6)6 : Sum  Inputs=+|-  RndMeth=Nearest  SaturateOnIntegerOverflow=on  OutDataTypeStr=Inherit: Same as first input
  densum1(7)7 : Sum  Inputs=+|-  RndMeth=Nearest  SaturateOnIntegerOverflow=on  OutDataTypeStr=Inherit: Same as first input
  densum2(1)1 : Sum  Inputs=+|-  RndMeth=Nearest  SaturateOnIntegerOverflow=on  OutDataTypeStr=Inherit: Same as first input
  densum2(2)2 : Sum  Inputs=+|-  RndMeth=Nearest  SaturateOnIntegerOverflow=on  OutDataTypeStr=Inherit: Same as first input
  densum2(3)3 : Sum  Inputs=+|-  RndMeth=Nearest  SaturateOnIntegerOverflow=on  OutDataTypeStr=Inherit: Same as first input
  densum2(4)4 : Sum  Inputs=+|-  RndMeth=Nearest  SaturateOnIntegerOverflow=on  OutDataTypeStr=Inherit: Same as first input
  densum2(5)5 : Sum  Inputs=+|-  RndMeth=Nearest  SaturateOnIntegerOverflow=on  OutDataTypeStr=Inherit: Same as first input
  densum2(6)6 : Sum  Inputs=+|-  RndMeth=Nearest  SaturateOnIntegerOverflow=on  OutDataTypeStr=Inherit: Same as first input
  densum2(7)7 : Sum  Inputs=+|-  RndMeth=Nearest  SaturateOnIntegerOverflow=on  OutDataTypeStr=Inherit: Same as first input
  gain1(1)(1) : Gain  Gain=-0.042904944031649322  ParamDataTypeStr=double  RndMeth=Nearest  SaturateOnIntegerOverflow=on  OutDataTypeStr=Inherit: Same as input
  gain1(2)(2) : Gain  Gain=-0.15851285525238301  ParamDataTypeStr=double  RndMeth=Nearest  SaturateOnIntegerOverflow=on  OutDataTypeStr=Inherit: Same as input
  gain1(3)(3) : Gain  Gain=-0.31578769921985456  ParamDataTypeStr=double  RndMeth=Nearest  SaturateOnIntegerOverflow=on  OutDataTypeStr=Inherit: Same as input
  gain1(4)(4) : Gain  Gain=-0.48276583745472768  ParamDataTypeStr=double  RndMeth=Nearest  SaturateOnIntegerOverflow=on  OutDataTypeStr=Inherit: Same as input
  gain1(5)(5) : Gain  Gain=-0.63887449831122922  ParamDataTypeStr=double  RndMeth=Nearest  SaturateOnIntegerOverflow=on  OutDataTypeStr=Inherit: Same as input
  gain1(6)(6) : Gain  Gain=-0.77777288596986116  ParamDataTypeStr=double  RndMeth=Nearest  SaturateOnIntegerOverflow=on  OutDataTypeStr=Inherit: Same as input
  gain1(7)(7) : Gain  Gain=-0.90465457400821292  ParamDataTypeStr=double  RndMeth=Nearest  SaturateOnIntegerOverflow=on  OutDataTypeStr=Inherit: Same as input
  gain2(1)(1) : Gain  Gain=0  ParamDataTypeStr=double  RndMeth=Nearest  SaturateOnIntegerOverflow=on  OutDataTypeStr=Inherit: Same as input
  gain2(2)(2) : Gain  Gain=0  ParamDataTypeStr=double  RndMeth=Nearest  SaturateOnIntegerOverflow=on  OutDataTypeStr=Inherit: Same as input
  gain2(3)(3) : Gain  Gain=0  ParamDataTypeStr=double  RndMeth=Nearest  SaturateOnIntegerOverflow=on  OutDataTypeStr=Inherit: Same as input
  gain2(4)(4) : Gain  Gain=0  ParamDataTypeStr=double  RndMeth=Nearest  SaturateOnIntegerOverflow=on  OutDataTypeStr=Inherit: Same as input
  gain2(5)(5) : Gain  Gain=0  ParamDataTypeStr=double  RndMeth=Nearest  SaturateOnIntegerOverflow=on  OutDataTypeStr=Inherit: Same as input
  gain2(6)(6) : Gain  Gain=0  ParamDataTypeStr=double  RndMeth=Nearest  SaturateOnIntegerOverflow=on  OutDataTypeStr=Inherit: Same as input
  gain2(7)(7) : Gain  Gain=0  ParamDataTypeStr=double  RndMeth=Nearest  SaturateOnIntegerOverflow=on  OutDataTypeStr=Inherit: Same as input
  numsum1(1)1 : Sum  Inputs=++|  RndMeth=Nearest  SaturateOnIntegerOverflow=on  OutDataTypeStr=Inherit: Same as first input
  numsum1(2)2 : Sum  Inputs=|++  RndMeth=Nearest  SaturateOnIntegerOverflow=on  OutDataTypeStr=Inherit: Same as first input
  numsum1(3)3 : Sum  Inputs=++|  RndMeth=Nearest  SaturateOnIntegerOverflow=on  OutDataTypeStr=Inherit: Same as first input
  numsum1(4)4 : Sum  Inputs=|++  RndMeth=Nearest  SaturateOnIntegerOverflow=on  OutDataTypeStr=Inherit: Same as first input
  numsum1(5)5 : Sum  Inputs=++|  RndMeth=Nearest  SaturateOnIntegerOverflow=on  OutDataTypeStr=Inherit: Same as first input
  numsum1(6)6 : Sum  Inputs=|++  RndMeth=Nearest  SaturateOnIntegerOverflow=on  OutDataTypeStr=Inherit: Same as first input
  numsum1(7)7 : Sum  Inputs=++|  RndMeth=Nearest  SaturateOnIntegerOverflow=on  OutDataTypeStr=Inherit: Same as first input
  numsum2(1)1 : Sum  Inputs=++|  RndMeth=Nearest  SaturateOnIntegerOverflow=on  OutDataTypeStr=Inherit: Same as first input
  numsum2(2)2 : Sum  Inputs=|++  RndMeth=Nearest  SaturateOnIntegerOverflow=on  OutDataTypeStr=Inherit: Same as first input
  numsum2(3)3 : Sum  Inputs=++|  RndMeth=Nearest  SaturateOnIntegerOverflow=on  OutDataTypeStr=Inherit: Same as first input
  numsum2(4)4 : Sum  Inputs=|++  RndMeth=Nearest  SaturateOnIntegerOverflow=on  OutDataTypeStr=Inherit: Same as first input
  numsum2(5)5 : Sum  Inputs=++|  RndMeth=Nearest  SaturateOnIntegerOverflow=on  OutDataTypeStr=Inherit: Same as first input
  numsum2(6)6 : Sum  Inputs=|++  RndMeth=Nearest  SaturateOnIntegerOverflow=on  OutDataTypeStr=Inherit: Same as first input
  numsum2(7)7 : Sum  Inputs=++|  RndMeth=Nearest  SaturateOnIntegerOverflow=on  OutDataTypeStr=Inherit: Same as first input
  output : Outport
  wires:
  delay1(1)1/1 -> delay2(1)1/1, densum2(1)1/1
  delay2(1)1/1 -> numsum1(1)1/2
  densum1(1)1/1 -> gain1(1)(1)/1
  gain1(1)(1)/1 -> numsum1(1)1/1
  numsum1(1)1/1 -> numsum2(1)1/2
  densum2(1)1/1 -> gain2(1)(1)/1
  gain2(1)(1)/1 -> numsum2(1)1/1
  numsum2(1)1/1 -> delay1(2)2/1, densum1(2)2/1
  Input/1 -> delay1(1)1/1, densum1(1)1/1
  delay1(2)2/1 -> delay2(2)2/1, densum2(2)2/1, densum2(1)1/2
  delay2(2)2/1 -> numsum1(2)2/1, densum1(1)1/2
  densum1(2)2/1 -> gain1(2)(2)/1
  gain1(2)(2)/1 -> numsum1(2)2/2
  numsum1(2)2/1 -> numsum2(2)2/1
  densum2(2)2/1 -> gain2(2)(2)/1
  gain2(2)(2)/1 -> numsum2(2)2/2
  numsum2(2)2/1 -> delay1(3)3/1, densum1(3)3/1
  delay1(3)3/1 -> delay2(3)3/1, densum2(3)3/1, densum2(2)2/2
  delay2(3)3/1 -> numsum1(3)3/2, densum1(2)2/2
  densum1(3)3/1 -> gain1(3)(3)/1
  gain1(3)(3)/1 -> numsum1(3)3/1
  numsum1(3)3/1 -> numsum2(3)3/2
  densum2(3)3/1 -> gain2(3)(3)/1
  gain2(3)(3)/1 -> numsum2(3)3/1
  numsum2(3)3/1 -> delay1(4)4/1, densum1(4)4/1
  delay1(4)4/1 -> delay2(4)4/1, densum2(4)4/1, densum2(3)3/2
  delay2(4)4/1 -> numsum1(4)4/1, densum1(3)3/2
  densum1(4)4/1 -> gain1(4)(4)/1
  gain1(4)(4)/1 -> numsum1(4)4/2
  numsum1(4)4/1 -> numsum2(4)4/1
  densum2(4)4/1 -> gain2(4)(4)/1
  gain2(4)(4)/1 -> numsum2(4)4/2
  numsum2(4)4/1 -> delay1(5)5/1, densum1(5)5/1
  delay1(5)5/1 -> delay2(5)5/1, densum2(5)5/1, densum2(4)4/2
  delay2(5)5/1 -> numsum1(5)5/2, densum1(4)4/2
  densum1(5)5/1 -> gain1(5)(5)/1
  gain1(5)(5)/1 -> numsum1(5)5/1
  numsum1(5)5/1 -> numsum2(5)5/2
  densum2(5)5/1 -> gain2(5)(5)/1
  gain2(5)(5)/1 -> numsum2(5)5/1
  numsum2(5)5/1 -> delay1(6)6/1, densum1(6)6/1
  delay1(6)6/1 -> delay2(6)6/1, densum2(6)6/1, densum2(5)5/2
  delay2(6)6/1 -> numsum1(6)6/1, densum1(5)5/2
  densum1(6)6/1 -> gain1(6)(6)/1
  gain1(6)(6)/1 -> numsum1(6)6/2
  numsum1(6)6/1 -> numsum2(6)6/1
  densum2(6)6/1 -> gain2(6)(6)/1
  gain2(6)(6)/1 -> numsum2(6)6/2
  numsum2(6)6/1 -> delay1(7)7/1, densum1(7)7/1
  delay1(7)7/1 -> delay2(7)7/1, densum2(7)7/1, densum2(6)6/2
  delay2(7)7/1 -> numsum1(7)7/2, densum1(6)6/2
  densum1(7)7/1 -> gain1(7)(7)/1
  gain1(7)(7)/1 -> numsum1(7)7/1
  numsum1(7)7/1 -> numsum2(7)7/2
  densum2(7)7/1 -> gain2(7)(7)/1
  gain2(7)(7)/1 -> numsum2(7)7/1
  numsum2(7)7/1 -> delay1(8)8/1, output/1
  delay1(8)8/1 -> delay2(8)8/1, densum2(7)7/2
  delay2(8)8/1 -> densum1(7)7/2

== system image_reject/Hilbert Filter1/Generated Filter Block/Stage1/Stage2/Stage2/Stage1 ==
  Input : Inport
  g(1) : Gain  Gain=-1  ParamDataTypeStr=double  RndMeth=Nearest  SaturateOnIntegerOverflow=on  OutDataTypeStr=Inherit: Same as input
  Output : Outport
  wires:
  Input/1 -> g(1)/1
  g(1)/1 -> Output/1

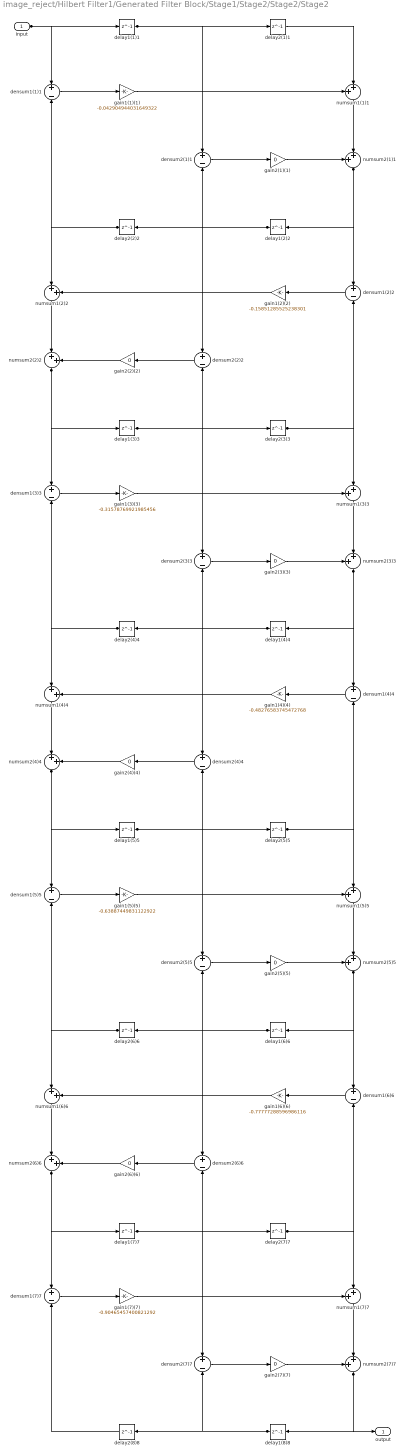
== system image_reject/Hilbert Filter1/Generated Filter Block/Stage1/Stage2/Stage2/Stage2 ==
  Input : Inport
  delay1(1)1 : Delay  DelayLength=1  InitialCondition=0
  delay1(2)2 : Delay  DelayLength=1  InitialCondition=0
  delay1(3)3 : Delay  DelayLength=1  InitialCondition=0
  delay1(4)4 : Delay  DelayLength=1  InitialCondition=0
  delay1(5)5 : Delay  DelayLength=1  InitialCondition=0
  delay1(6)6 : Delay  DelayLength=1  InitialCondition=0
  delay1(7)7 : Delay  DelayLength=1  InitialCondition=0
  delay1(8)8 : Delay  DelayLength=1  InitialCondition=0
  delay2(1)1 : Delay  DelayLength=1  InitialCondition=0
  delay2(2)2 : Delay  DelayLength=1  InitialCondition=0
  delay2(3)3 : Delay  DelayLength=1  InitialCondition=0
  delay2(4)4 : Delay  DelayLength=1  InitialCondition=0
  delay2(5)5 : Delay  DelayLength=1  InitialCondition=0
  delay2(6)6 : Delay  DelayLength=1  InitialCondition=0
  delay2(7)7 : Delay  DelayLength=1  InitialCondition=0
  delay2(8)8 : Delay  DelayLength=1  InitialCondition=0
  densum1(1)1 : Sum  Inputs=+|-  RndMeth=Nearest  SaturateOnIntegerOverflow=on  OutDataTypeStr=Inherit: Same as first input
  densum1(2)2 : Sum  Inputs=+|-  RndMeth=Nearest  SaturateOnIntegerOverflow=on  OutDataTypeStr=Inherit: Same as first input
  densum1(3)3 : Sum  Inputs=+|-  RndMeth=Nearest  SaturateOnIntegerOverflow=on  OutDataTypeStr=Inherit: Same as first input
  densum1(4)4 : Sum  Inputs=+|-  RndMeth=Nearest  SaturateOnIntegerOverflow=on  OutDataTypeStr=Inherit: Same as first input
  densum1(5)5 : Sum  Inputs=+|-  RndMeth=Nearest  SaturateOnIntegerOverflow=on  OutDataTypeStr=Inherit: Same as first input
  densum1(6)6 : Sum  Inputs=+|-  RndMeth=Nearest  SaturateOnIntegerOverflow=on  OutDataTypeStr=Inherit: Same as first input
  densum1(7)7 : Sum  Inputs=+|-  RndMeth=Nearest  SaturateOnIntegerOverflow=on  OutDataTypeStr=Inherit: Same as first input
  densum2(1)1 : Sum  Inputs=+|-  RndMeth=Nearest  SaturateOnIntegerOverflow=on  OutDataTypeStr=Inherit: Same as first input
  densum2(2)2 : Sum  Inputs=+|-  RndMeth=Nearest  SaturateOnIntegerOverflow=on  OutDataTypeStr=Inherit: Same as first input
  densum2(3)3 : Sum  Inputs=+|-  RndMeth=Nearest  SaturateOnIntegerOverflow=on  OutDataTypeStr=Inherit: Same as first input
  densum2(4)4 : Sum  Inputs=+|-  RndMeth=Nearest  SaturateOnIntegerOverflow=on  OutDataTypeStr=Inherit: Same as first input
  densum2(5)5 : Sum  Inputs=+|-  RndMeth=Nearest  SaturateOnIntegerOverflow=on  OutDataTypeStr=Inherit: Same as first input
  densum2(6)6 : Sum  Inputs=+|-  RndMeth=Nearest  SaturateOnIntegerOverflow=on  OutDataTypeStr=Inherit: Same as first input
  densum2(7)7 : Sum  Inputs=+|-  RndMeth=Nearest  SaturateOnIntegerOverflow=on  OutDataTypeStr=Inherit: Same as first input
  gain1(1)(1) : Gain  Gain=-0.042904944031649322  ParamDataTypeStr=double  RndMeth=Nearest  SaturateOnIntegerOverflow=on  OutDataTypeStr=Inherit: Same as input
  gain1(2)(2) : Gain  Gain=-0.15851285525238301  ParamDataTypeStr=double  RndMeth=Nearest  SaturateOnIntegerOverflow=on  OutDataTypeStr=Inherit: Same as input
  gain1(3)(3) : Gain  Gain=-0.31578769921985456  ParamDataTypeStr=double  RndMeth=Nearest  SaturateOnIntegerOverflow=on  OutDataTypeStr=Inherit: Same as input
  gain1(4)(4) : Gain  Gain=-0.48276583745472768  ParamDataTypeStr=double  RndMeth=Nearest  SaturateOnIntegerOverflow=on  OutDataTypeStr=Inherit: Same as input
  gain1(5)(5) : Gain  Gain=-0.63887449831122922  ParamDataTypeStr=double  RndMeth=Nearest  SaturateOnIntegerOverflow=on  OutDataTypeStr=Inherit: Same as input
  gain1(6)(6) : Gain  Gain=-0.77777288596986116  ParamDataTypeStr=double  RndMeth=Nearest  SaturateOnIntegerOverflow=on  OutDataTypeStr=Inherit: Same as input
  gain1(7)(7) : Gain  Gain=-0.90465457400821292  ParamDataTypeStr=double  RndMeth=Nearest  SaturateOnIntegerOverflow=on  OutDataTypeStr=Inherit: Same as input
  gain2(1)(1) : Gain  Gain=0  ParamDataTypeStr=double  RndMeth=Nearest  SaturateOnIntegerOverflow=on  OutDataTypeStr=Inherit: Same as input
  gain2(2)(2) : Gain  Gain=0  ParamDataTypeStr=double  RndMeth=Nearest  SaturateOnIntegerOverflow=on  OutDataTypeStr=Inherit: Same as input
  gain2(3)(3) : Gain  Gain=0  ParamDataTypeStr=double  RndMeth=Nearest  SaturateOnIntegerOverflow=on  OutDataTypeStr=Inherit: Same as input
  gain2(4)(4) : Gain  Gain=0  ParamDataTypeStr=double  RndMeth=Nearest  SaturateOnIntegerOverflow=on  OutDataTypeStr=Inherit: Same as input
  gain2(5)(5) : Gain  Gain=0  ParamDataTypeStr=double  RndMeth=Nearest  SaturateOnIntegerOverflow=on  OutDataTypeStr=Inherit: Same as input
  gain2(6)(6) : Gain  Gain=0  ParamDataTypeStr=double  RndMeth=Nearest  SaturateOnIntegerOverflow=on  OutDataTypeStr=Inherit: Same as input
  gain2(7)(7) : Gain  Gain=0  ParamDataTypeStr=double  RndMeth=Nearest  SaturateOnIntegerOverflow=on  OutDataTypeStr=Inherit: Same as input
  numsum1(1)1 : Sum  Inputs=++|  RndMeth=Nearest  SaturateOnIntegerOverflow=on  OutDataTypeStr=Inherit: Same as first input
  numsum1(2)2 : Sum  Inputs=|++  RndMeth=Nearest  SaturateOnIntegerOverflow=on  OutDataTypeStr=Inherit: Same as first input
  numsum1(3)3 : Sum  Inputs=++|  RndMeth=Nearest  SaturateOnIntegerOverflow=on  OutDataTypeStr=Inherit: Same as first input
  numsum1(4)4 : Sum  Inputs=|++  RndMeth=Nearest  SaturateOnIntegerOverflow=on  OutDataTypeStr=Inherit: Same as first input
  numsum1(5)5 : Sum  Inputs=++|  RndMeth=Nearest  SaturateOnIntegerOverflow=on  OutDataTypeStr=Inherit: Same as first input
  numsum1(6)6 : Sum  Inputs=|++  RndMeth=Nearest  SaturateOnIntegerOverflow=on  OutDataTypeStr=Inherit: Same as first input
  numsum1(7)7 : Sum  Inputs=++|  RndMeth=Nearest  SaturateOnIntegerOverflow=on  OutDataTypeStr=Inherit: Same as first input
  numsum2(1)1 : Sum  Inputs=++|  RndMeth=Nearest  SaturateOnIntegerOverflow=on  OutDataTypeStr=Inherit: Same as first input
  numsum2(2)2 : Sum  Inputs=|++  RndMeth=Nearest  SaturateOnIntegerOverflow=on  OutDataTypeStr=Inherit: Same as first input
  numsum2(3)3 : Sum  Inputs=++|  RndMeth=Nearest  SaturateOnIntegerOverflow=on  OutDataTypeStr=Inherit: Same as first input
  numsum2(4)4 : Sum  Inputs=|++  RndMeth=Nearest  SaturateOnIntegerOverflow=on  OutDataTypeStr=Inherit: Same as first input
  numsum2(5)5 : Sum  Inputs=++|  RndMeth=Nearest  SaturateOnIntegerOverflow=on  OutDataTypeStr=Inherit: Same as first input
  numsum2(6)6 : Sum  Inputs=|++  RndMeth=Nearest  SaturateOnIntegerOverflow=on  OutDataTypeStr=Inherit: Same as first input
  numsum2(7)7 : Sum  Inputs=++|  RndMeth=Nearest  SaturateOnIntegerOverflow=on  OutDataTypeStr=Inherit: Same as first input
  output : Outport
  wires:
  delay1(1)1/1 -> delay2(1)1/1, densum2(1)1/1
  delay2(1)1/1 -> numsum1(1)1/2
  densum1(1)1/1 -> gain1(1)(1)/1
  gain1(1)(1)/1 -> numsum1(1)1/1
  numsum1(1)1/1 -> numsum2(1)1/2
  densum2(1)1/1 -> gain2(1)(1)/1
  gain2(1)(1)/1 -> numsum2(1)1/1
  numsum2(1)1/1 -> delay1(2)2/1, densum1(2)2/1
  Input/1 -> delay1(1)1/1, densum1(1)1/1
  delay1(2)2/1 -> delay2(2)2/1, densum2(2)2/1, densum2(1)1/2
  delay2(2)2/1 -> numsum1(2)2/1, densum1(1)1/2
  densum1(2)2/1 -> gain1(2)(2)/1
  gain1(2)(2)/1 -> numsum1(2)2/2
  numsum1(2)2/1 -> numsum2(2)2/1
  densum2(2)2/1 -> gain2(2)(2)/1
  gain2(2)(2)/1 -> numsum2(2)2/2
  numsum2(2)2/1 -> delay1(3)3/1, densum1(3)3/1
  delay1(3)3/1 -> delay2(3)3/1, densum2(3)3/1, densum2(2)2/2
  delay2(3)3/1 -> numsum1(3)3/2, densum1(2)2/2
  densum1(3)3/1 -> gain1(3)(3)/1
  gain1(3)(3)/1 -> numsum1(3)3/1
  numsum1(3)3/1 -> numsum2(3)3/2
  densum2(3)3/1 -> gain2(3)(3)/1
  gain2(3)(3)/1 -> numsum2(3)3/1
  numsum2(3)3/1 -> delay1(4)4/1, densum1(4)4/1
  delay1(4)4/1 -> delay2(4)4/1, densum2(4)4/1, densum2(3)3/2
  delay2(4)4/1 -> numsum1(4)4/1, densum1(3)3/2
  densum1(4)4/1 -> gain1(4)(4)/1
  gain1(4)(4)/1 -> numsum1(4)4/2
  numsum1(4)4/1 -> numsum2(4)4/1
  densum2(4)4/1 -> gain2(4)(4)/1
  gain2(4)(4)/1 -> numsum2(4)4/2
  numsum2(4)4/1 -> delay1(5)5/1, densum1(5)5/1
  delay1(5)5/1 -> delay2(5)5/1, densum2(5)5/1, densum2(4)4/2
  delay2(5)5/1 -> numsum1(5)5/2, densum1(4)4/2
  densum1(5)5/1 -> gain1(5)(5)/1
  gain1(5)(5)/1 -> numsum1(5)5/1
  numsum1(5)5/1 -> numsum2(5)5/2
  densum2(5)5/1 -> gain2(5)(5)/1
  gain2(5)(5)/1 -> numsum2(5)5/1
  numsum2(5)5/1 -> delay1(6)6/1, densum1(6)6/1
  delay1(6)6/1 -> delay2(6)6/1, densum2(6)6/1, densum2(5)5/2
  delay2(6)6/1 -> numsum1(6)6/1, densum1(5)5/2
  densum1(6)6/1 -> gain1(6)(6)/1
  gain1(6)(6)/1 -> numsum1(6)6/2
  numsum1(6)6/1 -> numsum2(6)6/1
  densum2(6)6/1 -> gain2(6)(6)/1
  gain2(6)(6)/1 -> numsum2(6)6/2
  numsum2(6)6/1 -> delay1(7)7/1, densum1(7)7/1
  delay1(7)7/1 -> delay2(7)7/1, densum2(7)7/1, densum2(6)6/2
  delay2(7)7/1 -> numsum1(7)7/2, densum1(6)6/2
  densum1(7)7/1 -> gain1(7)(7)/1
  gain1(7)(7)/1 -> numsum1(7)7/1
  numsum1(7)7/1 -> numsum2(7)7/2
  densum2(7)7/1 -> gain2(7)(7)/1
  gain2(7)(7)/1 -> numsum2(7)7/1
  numsum2(7)7/1 -> delay1(8)8/1, output/1
  delay1(8)8/1 -> delay2(8)8/1, densum2(7)7/2
  delay2(8)8/1 -> densum1(7)7/2
